simulink model "slx_Pendulum_Continuo"  (R2023a)
settings: Solver=ode45  StartTime=0  StopTime=simulation_T_f  MaxStep=MaxStep  RelTol=RelTol  AbsTol=1e-6
values from neighbouring files (symbols this model uses):
  A_CTRL_angle = f_KR_angle_LTI.A    [Tesi_DiscretoCascade.m]    (also in tesi_sperimentale.m)
  A_CTRL_position = f_KR_position_LTI.A    [Tesi_DiscretoCascade.m]    (also in tesi_sperimentale.m)
  B_CTRL_angle = f_KR_angle_LTI.B    [Tesi_DiscretoCascade.m]    (also in tesi_sperimentale.m)
  B_CTRL_position = f_KR_position_LTI.B    [Tesi_DiscretoCascade.m]    (also in tesi_sperimentale.m)
  C_CTRL_angle = f_KR_angle_LTI.C    [Tesi_DiscretoCascade.m]    (also in tesi_sperimentale.m)
  C_CTRL_position = f_KR_position_LTI.C    [Tesi_DiscretoCascade.m]    (also in tesi_sperimentale.m)
  D_CTRL_angle = f_KR_angle_LTI.D    [Tesi_DiscretoCascade.m]    (also in tesi_sperimentale.m)
  D_CTRL_position = f_KR_position_LTI.D    [Tesi_DiscretoCascade.m]    (also in tesi_sperimentale.m)
  init_omega0 = 0    [Tesi_DiscretoCascade.m]    (also in tesi_sperimentale.m)
  init_positionRef = 0    [Tesi_DiscretoCascade.m]    (also in tesi_sperimentale.m)
  init_theta0 = pi/12    (= 0.261799387799)    [Tesi_DiscretoCascade.m]    (also in tesi_sperimentale.m)
  init_thetaRef = 0    [Tesi_DiscretoCascade.m]    (also in tesi_sperimentale.m)
  init_v0 = 0    [Tesi_DiscretoCascade.m]    (also in tesi_sperimentale.m)
  init_x0 = -3    [Tesi_DiscretoCascade.m]    (also in tesi_sperimentale.m = -5)
  p_b = 0.1    [Tesi_DiscretoCascade.m]    (also in tesi_sperimentale.m)
  p_g = 9.81    [Tesi_DiscretoCascade.m]    (also in tesi_sperimentale.m)
  p_Ja = (1/12)*p_ma*p_l^2    (= 0.0019575)    [Tesi_DiscretoCascade.m]    (also in tesi_sperimentale.m)
  p_Jb = 0    [Tesi_DiscretoCascade.m]    (also in tesi_sperimentale.m)
  p_k = 0    [Tesi_DiscretoCascade.m]    (also in tesi_sperimentale.m)
  p_l = 0.45    [Tesi_DiscretoCascade.m]    (also in tesi_sperimentale.m)
  p_M = 0.61    [Tesi_DiscretoCascade.m]    (also in tesi_sperimentale.m)
  p_ma = 0.116    [Tesi_DiscretoCascade.m]    (also in tesi_sperimentale.m)
  p_mb = 0.05    [Tesi_DiscretoCascade.m]    (also in tesi_sperimentale.m)
Description:
  | Inverted Pendulum with Animation
  | 
  | This example shows how to model an inverted pendulum.  The animation is created using MATLAB(R) Handle Graphics(R).  The animation block is a masked
  | S-function.  For more information, use the context menu to look under the Animation block's mask
  | and open the S-function for editing.
settings Model: Creator=The MathWorks, Inc.  LastModifiedBy=admin
settings SolverCC: AutoScaleAbsTol=off  AlgebraicLoopSolver=TrustRegion
settings DataIOCC: ExternalInput=[]  InitialState=[]  SaveFormat=Array  SaveOutput=off  SaveTime=off  ReturnWorkspaceOutputs=off
settings OptimizationCC: BlockReduction=off  BooleanDataType=off  ReuseModelBlockBuffer=off  ExpressionDepthLimit=2147483647  InitFltsAndDblsToZero=on  LifeSpan=inf
settings DebuggingCC: SaveWithParameterizedLinksMsg=none  UnderspecifiedInitializationDetection=Classic  MergeDetectMultiDrivingBlocksExec=none  SignalResolutionControl=TryResolveAllWithWarning  MultiTaskDSMMsg=warning  MultiTaskCondExecSysMsg=none  SigSpecEnsureSampleTimeMsg=none  FcnCallInpInsideContextMsg=warning  UnconnectedInputMsg=warning  UnconnectedOutputMsg=warning  UnconnectedLineMsg=warning  StateNameClashWarn=warning  SFUnexpectedBacktrackingDiag=warning  SFNoUnconditionalDefaultTransitionDiag=warning  SFExecutionAtInitializationDiag=none  ArithmeticOperatorsInVariantConditions=warning
settings HardwareCC: ProdBitPerPointer=32  ProdBitPerSizeT=32  ProdBitPerPtrDiffT=32  ProdLargestAtomicFloat=None  ProdIntDivRoundTo=Undefined  ProdEndianess=Unspecified  ProdWordSize=32  ProdHWDeviceType=32-bit Generic  TargetUnknown=on
settings ModelReferenceCC: EnableRefExpFcnMdlSchedulingChecks=on  PropagateSignalLabelsOutOfModel=off
settings SFSimCC: SimUseLocalCustomCode=off  CustomCodeUndefinedFunction=UseInterfaceOnly
settings RTWCC: RTWUseLocalCustomCode=off
settings CodeAppCC: StateflowObjectComments=on
settings GRTTargetCC: TargetFcnLib=ansi_tfl_tmw.mat  TargetLangStandard=C89/C90 (ANSI)  CombineOutputUpdateFcns=off  GRTInterface=on
settings ConfigComp: CovMetricSettings=dw  CovSaveCumulativeToWorkspaceVar=on  CovSaveSingleToWorkspaceVar=on  CovExternalEMLEnable=off

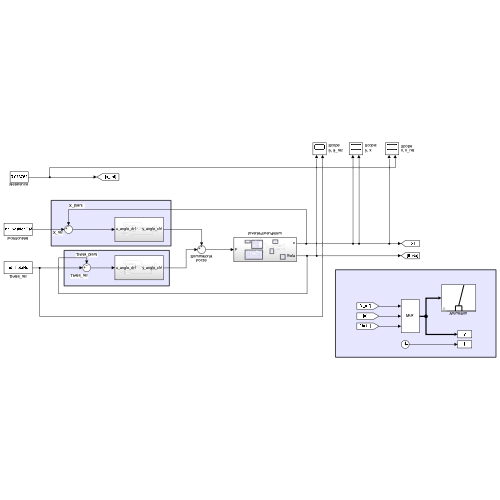
[thumbnail: Simulink's stored preview of the top-level diagram]
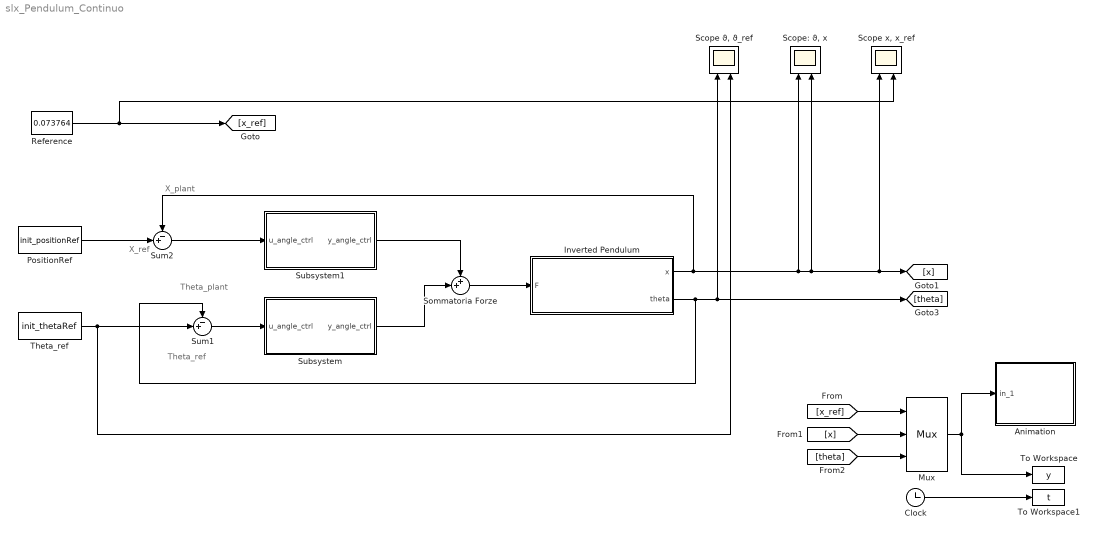
== system slx_Pendulum_Continuo ==
  note: Theta_plant
  note: Theta_ref
  note: X_plant
  note: X_ref
  Animation : Subsystem  mask(Pendulum plot){RefBlock=Reference}
      mask prompts: RefBlock "DC reference signal block name:"
      mask help: Pendulum plot
      mask Help: Pendulum animation function using Handle graphics.
      mask Display: plot([-10 10],[0 0],[-2 -2 2 2],[0 1 1 0],[0 3],[1 5])
  Clock : Clock
  Inverted Pendulum : Subsystem
  Mux : Mux  Inputs=3
  PositionRef : Constant  Value=init_positionRef
  Reference : Constant  Value=0.073764
  "Scope x, x_ref" : Scope  NumInputPorts=2
  "Scope ϑ, ϑ_ref" : Scope  NumInputPorts=2
  "Scope: ϑ, x" : Scope  NumInputPorts=2
  Sommatoria Forze : Sum  Inputs=++|
  Subsystem : Subsystem
  Subsystem1 : Subsystem
  Sum1 : Sum  Inputs=-+|
  Sum2 : Sum  Inputs=-+|
  Theta_ref : Constant  Value=init_thetaRef
  To Workspace : ToWorkspace  VariableName=y  SampleTime=0.02
  To Workspace1 : ToWorkspace  VariableName=t  SampleTime=0.02
  wires:
  Reference/1 -> [x_ref], "Scope x, x_ref"/2
  [x_ref] -> Mux/1
  [x] -> Mux/2
  [theta] -> Mux/3
  Mux/1 -> To Workspace/1, Animation/1(in_1)
  Clock/1 -> To Workspace1/1
  Inverted Pendulum/1(x) -> "Scope: ϑ, x"/1, "Scope x, x_ref"/1, [x], "Scope: ϑ, x"/2, Sum2/1
  Inverted Pendulum/2(theta) -> "Scope ϑ, ϑ_ref"/1, [theta], Sum1/1
  Theta_ref/1 -> Sum1/2, "Scope ϑ, ϑ_ref"/2
  Sum1/1 -> Subsystem/1(u_angle_ctrl)
  Subsystem/1(y_angle_ctrl) -> Sommatoria Forze/2
  Sommatoria Forze/1 -> Inverted Pendulum/1(F)
  PositionRef/1 -> Sum2/2
  Sum2/1 -> Subsystem1/1(u_angle_ctrl)
  Subsystem1/1(y_angle_ctrl) -> Sommatoria Forze/1

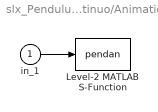
== system slx_Pendulum_Continuo/Animation ==
  in_1 : Inport
  Level-2 MATLAB S-Function : M-S-Function  FunctionName=pendan  Parameters=RefBlock
  wires:
  in_1/1 -> Level-2 MATLAB S-Function/1

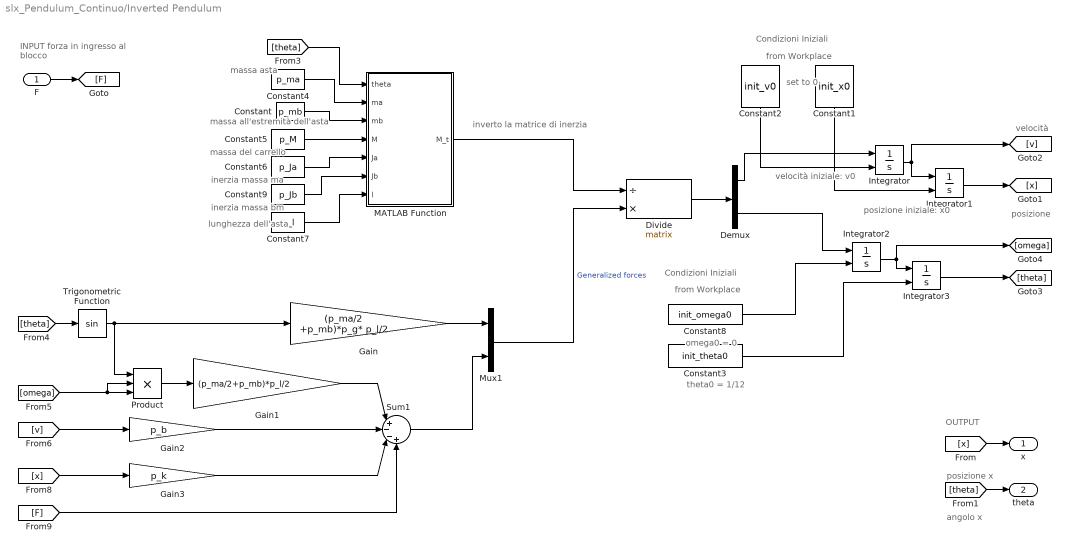
== system slx_Pendulum_Continuo/Inverted Pendulum ==
  note: from Workplace
  note: posizione x
  note: inverto la matrice di inerzia
  note: inerzia massa ma
  note: massa del carrello
  note: massa asta
  note: INPUT
      | forza in ingresso al blocco
  note: massa all'estremità
      | dell'asta
  note: inerzia massa bm
  note: lunghezza dell'asta
  note: OUTPUT
  note: angolo x
  note: theta0 = 1/12
  note: omega0 = 0
  note: from Workplace
  note: set to 0
  note: Condizioni Iniziali
  note: velocità
  note: posizione
  note: Condizioni Iniziali
  note: velocità iniziale: v0
  note: posizione iniziale: x0
  F : Inport
  Constant : Constant  Value=p_mb
  Constant1 : Constant  Value=init_x0
  Constant2 : Constant  Value=init_v0
  Constant3 : Constant  Value=init_theta0
  Constant4 : Constant  Value=p_ma
  Constant5 : Constant  Value=p_M
  Constant6 : Constant  Value=p_Ja
  Constant7 : Constant  Value=p_l
  Constant8 : Constant  Value=init_omega0
  Constant9 : Constant  Value=p_Jb
  Demux : Demux  Outputs=2
  Divide : Product  Inputs=/*  Multiplication=Matrix(*)
  Gain : Gain  Gain=(p_ma/2 +p_mb)*p_g* p_l/2
  Gain1 : Gain  Gain=(p_ma/2+p_mb)*p_l/2
  Gain2 : Gain  Gain=p_b
  Gain3 : Gain  Gain=p_k
  Integrator : Integrator  InitialConditionSource=external
  Integrator1 : Integrator  InitialConditionSource=external
  Integrator2 : Integrator  InitialConditionSource=external
  Integrator3 : Integrator  InitialConditionSource=external  WrapState=on
  MATLAB Function : MATLAB Function  TreatAsAtomicUnit=on
  Mux1 : Mux  Inputs=2
  Product : Product  Inputs=3
  Sum1 : Sum  Inputs=|+--+
  Trigonometric Function : Trigonometry
  x : Outport
  theta : Outport  Port=2
  wires:
  Integrator/1 -> [v], Integrator1/1
  Integrator3/1 -> [theta]
  [omega] -> Product/2, Product/3
  Integrator1/1 -> [x]
  Integrator2/1 -> Integrator3/1, [omega]
  Divide/1 -> Demux/1
  Demux/2 -> Integrator2/1
  Gain2/1 -> Sum1/2
  Sum1/1 -> Mux1/2
  [theta] -> Trigonometric Function/1
  Product/1 -> Gain1/1
  MATLAB Function/1(M_t) -> Divide/1
  Gain/1 -> Mux1/1
  Trigonometric Function/1 -> Gain/1, Product/1
  Mux1/1 -> Divide/2  "Generalized forces"
  [F] -> Sum1/4
  Gain1/1 -> Sum1/1
  Constant2/1 -> Integrator/2
  Constant3/1 -> Integrator3/2
  [x] -> Gain3/1
  Demux/1 -> Integrator/1
  Gain3/1 -> Sum1/3
  [v] -> Gain2/1
  Constant1/1 -> Integrator1/2
  F/1 -> [F]
  [x] -> x/1
  [theta] -> theta/1
  Constant8/1 -> Integrator2/2
  [theta] -> MATLAB Function/1(theta)
  Constant4/1 -> MATLAB Function/2(ma)
  Constant5/1 -> MATLAB Function/4(M)
  Constant/1 -> MATLAB Function/3(mb)
  Constant6/1 -> MATLAB Function/5(Ja)
  Constant9/1 -> MATLAB Function/6(Jb)
  Constant7/1 -> MATLAB Function/7(l)

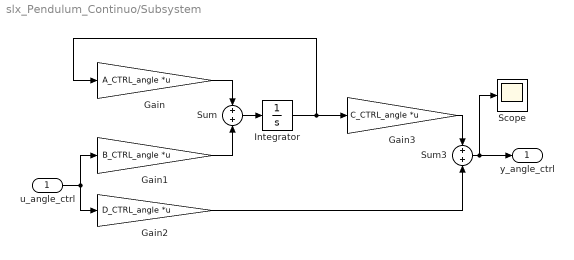
== system slx_Pendulum_Continuo/Subsystem ==
  u_angle_ctrl : Inport
  Gain : Gain  Gain=A_CTRL_angle  Multiplication=Matrix(K*u)
  Gain1 : Gain  Gain=B_CTRL_angle  Multiplication=Matrix(K*u)
  Gain2 : Gain  Gain=D_CTRL_angle  Multiplication=Matrix(K*u)
  Gain3 : Gain  Gain=C_CTRL_angle  Multiplication=Matrix(K*u)
  Integrator : Integrator
  Scope : Scope
  Sum : Sum
  Sum3 : Sum
  y_angle_ctrl : Outport
  wires:
  Integrator/1 -> Gain3/1, Gain/1
  Sum/1 -> Integrator/1
  Gain/1 -> Sum/1
  Sum3/1 -> y_angle_ctrl/1, Scope/1
  Gain3/1 -> Sum3/1
  Gain1/1 -> Sum/2
  Gain2/1 -> Sum3/2
  u_angle_ctrl/1 -> Gain2/1, Gain1/1

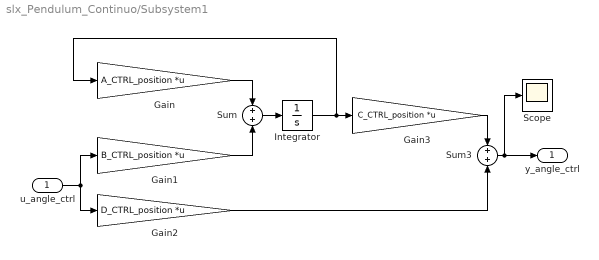
== system slx_Pendulum_Continuo/Subsystem1 ==
  u_angle_ctrl : Inport
  Gain : Gain  Gain=A_CTRL_position  Multiplication=Matrix(K*u)
  Gain1 : Gain  Gain=B_CTRL_position  Multiplication=Matrix(K*u)
  Gain2 : Gain  Gain=D_CTRL_position  Multiplication=Matrix(K*u)
  Gain3 : Gain  Gain=C_CTRL_position  Multiplication=Matrix(K*u)
  Integrator : Integrator
  Scope : Scope
  Sum : Sum
  Sum3 : Sum
  y_angle_ctrl : Outport
  wires:
  Integrator/1 -> Gain3/1, Gain/1
  Sum/1 -> Integrator/1
  Gain/1 -> Sum/1
  Sum3/1 -> y_angle_ctrl/1, Scope/1
  Gain3/1 -> Sum3/1
  Gain1/1 -> Sum/2
  Gain2/1 -> Sum3/2
  u_angle_ctrl/1 -> Gain2/1, Gain1/1

== matlab function slx_Pendulum_Continuo/Inverted Pendulum/MATLAB Function ==
  data: theta input; M_t output; ma input; mb input; M input; Ja input; Jb input; l input
function M_t = Inertia(theta, ma, mb, M, Ja, Jb, l)
%% Computation of the inertia matrix
M_t = [(ma/2+mb)*l*cos(theta) (ma/4+mb)*l^2+Ja+Jb;
            M+ma+mb (ma/2+mb)*l*cos(theta)];
